simulink model "PointProcessSimulationCont"  (R2013b)
settings: Solver=ode45  StartTime=0.0  StopTime=10  FixedStep=Ts  RelTol=1e-3
values from neighbouring files (symbols this model uses):
  mu = b    [Analysis.m]    (also in Covariate.m = mean(covObj); nspikeTrain.m = mean(ISI); nstColl.m = bVals)
  simTypeSelect = 0    [CIF.m]
  Ts = hist.Ts    [CIF.m]
undefined symbols (not defined in the file or in its folder): P, sampPerFrame, seed
libraries: cstblocks x3, dspsrcs4 x1
settings Model: Creator=Developer  LastModifiedBy=iahncajigas
settings OptimizationCC: ExpressionDepthLimit=2147483647
settings DebuggingCC: StateNameClashWarn=warning
settings HardwareCC: TargetBitPerLong=64  TargetBitPerPointer=64  TargetLongLongMode=on  TargetIntDivRoundTo=Zero  TargetEndianess=LittleEndian  TargetWordSize=64  TargetHWDeviceType=MATLAB Host  ProdEqTarget=off
settings RTWCC: ProcessScript=grt_make_rtw_hook  RTWCompilerOptimization=On
settings GRTTargetCC: CombineOutputUpdateFcns=off  GRTInterface=on

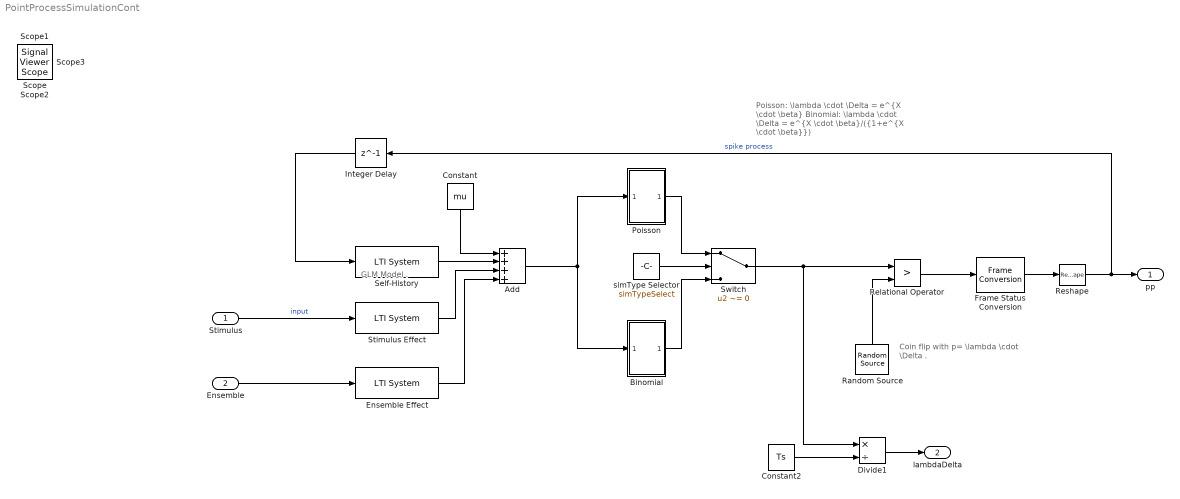
== system PointProcessSimulationCont ==
  note: GLM Model
      |
      |
      |
      |
      |
      |
      |
      |
      |
      |
      |
      |
      |
      |
      |
      |
      |
      |
      |
      |
      | .
  note: Coin flip with
      | p= \lambda \cdot \Delta
      |
      |
      |
      |
      |
      |
      |
      |
      |
      |
      | .
  note: Poisson:
      | \lambda \cdot \Delta = e^{X \cdot \beta}
      | Binomial:
      | \lambda \cdot \Delta = e^{X \cdot \beta}/({1+e^{X \cdot \beta}})
  Stimulus : Inport
  Ensemble : Inport  Port=2
  Add : Sum  Inputs=++++
  Binomial : Subsystem
  Constant : Constant  Value=mu
  Constant2 : Constant  Value=Ts
  Divide1 : Product  Inputs=*/
  Ensemble Effect : cstblocks/LTI System  sys=E  IC=[]
  Frame Status Conversion : FrameConversion  OutFrame=Sample-based
  Integer Delay : Delay  DelayLength=1
  Poisson : Subsystem
  Random Source : dspsrcs4/Random Source  SrcType=Uniform  NormMethod=Ziggurat  CltLength=12  MinVal=0  MaxVal=1  MeanVal=0  VarVal=1  RepMode=Not repeatable  rawSeed=seed  IsInherit=on  SampMode=Continuous  SampTime=Ts  SampFrame=dsp_sampFrame  DataType=Double  OutComplex=Real
  Relational Operator : RelationalOperator  Operator=>  OutDataTypeStr=float('double')  InputSameDT=on
  Reshape : Reshape  OutputDimensions=[sampPerFrame,max(length(P),length(seed))]
  Self-History : cstblocks/LTI System  sys=H  IC=[]
  Stimulus Effect : cstblocks/LTI System  sys=S  IC=[]
  Switch : Switch  Criteria=u2 ~= 0
  simType Selector : Constant  Value=simTypeSelect
  pp : Outport
  lambdaDelta : Outport  Port=2
  Scope{,1..3} (4 alike) : SignalViewerScope  IOType=viewer  RefreshTime=0.035000
      Scope settings: TimeRange=10
      Scope2 settings: SaveName=ScopeData2
      Scope3 settings: TimeRange=3.199999999999999  YMin=0.009803977272727278  YMax=0.02380397727272728  SaveName=ScopeData3
  wires:
  Constant/1 -> Add/1
  Self-History/1 -> Add/2
  Stimulus Effect/1 -> Add/3
  Add/1 -> Binomial/1(In1), Poisson/1(In1)
  Frame Status Conversion/1 -> Reshape/1
  Reshape/1 -> Integer Delay/1, pp/1  "spike process"
  Relational Operator/1 -> Frame Status Conversion/1
  Random Source/1 -> Relational Operator/2
  Stimulus/1 -> Stimulus Effect/1  "input"
  Integer Delay/1 -> Self-History/1
  Ensemble/1 -> Ensemble Effect/1
  Ensemble Effect/1 -> Add/4
  Constant2/1 -> Divide1/2
  Divide1/1 -> lambdaDelta/1
  simType Selector/1 -> Switch/2
  Binomial/1(Out1) -> Switch/3
  Switch/1 -> Relational Operator/1, Divide1/1
  Poisson/1(Out1) -> Switch/1

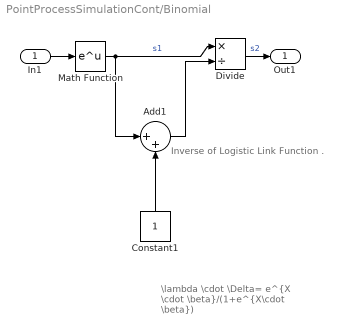
== system PointProcessSimulationCont/Binomial ==
  note: Inverse of Logistic Link Function
      |
      |
      |
      |
      |
      |
      |
      |
      |
      |
      | .
  note: \lambda \cdot \Delta= e^{X \cdot \beta}/(1+e^{X\cdot \beta})
  In1 : Inport
  Add1 : Sum  Inputs=|++
  Constant1 : Constant
  Divide : Product  Inputs=*/
  Math Function : Math  SaturateOnIntegerOverflow=on
  Out1 : Outport
  wires:
  Constant1/1 -> Add1/2
  Math Function/1 -> Add1/1, Divide/1  "s1"
  Add1/1 -> Divide/2
  Divide/1 -> Out1/1  "s2"
  In1/1 -> Math Function/1

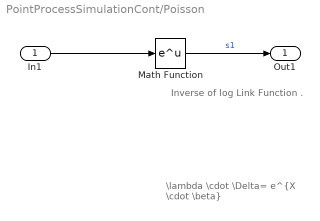
== system PointProcessSimulationCont/Poisson ==
  note: \lambda \cdot \Delta= e^{X \cdot \beta}
  note: Inverse of log Link Function
      |
      |
      |
      |
      |
      |
      | .
  In1 : Inport
  Math Function : Math  SaturateOnIntegerOverflow=on
  Out1 : Outport
  wires:
  In1/1 -> Math Function/1
  Math Function/1 -> Out1/1  "s1"
